simulink model "Final_EWASP_VC"  (R2022a)
settings: Solver=ode1  StartTime=0.0  StopTime=24*3600  FixedStep=10  RelTol=1e-3
values from neighbouring files (symbols this model uses):
  Aux_Threshold = 52    [Setup_Code_EWASP_VC.m]
  buildingAge = 2005    [Setup_Code_EWASP_VC.m]
  ceilingHeight = 2.4    [Setup_Code_EWASP_VC.m]
  conductiveHconnectMatrix = [ ... (first row only)    [Setup_Code_EWASP_VC.m]
  cRoofGreen = 100000    [Setup_Code_EWASP_VC.m]
  Defrost_After_Time = 30    [Setup_Code_EWASP_VC.m]
  DHWDemandProfile = occFreegainHotwaterElecTestPassiveOcc3(:,3)    [Setup_Code_EWASP_VC.m]
  Elec_Max = Elec_Max*(30/24.2)    [Setup_Code_EWASP_VC.m]
  Elec_Mid = Elec_Mid*(30/24.2)    [Setup_Code_EWASP_VC.m]
  Elec_Min = Elec_Min*(30/24.2)    [Setup_Code_EWASP_VC.m]
  ElecDemandProfile = occFreegainHotwaterElecTestPassiveOcc3(:,4)    [Setup_Code_EWASP_VC.m]
  ElecFixed = [Elec_Max(6,2) Elec_Max(6,4) Elec_Max(6,6) Elec_Max(6,7) ... (first row only)    [Setup_Code_EWASP_VC.m]
  floorOrCeilingArea = floorOrCeilingArea*1.15    [Setup_Code_EWASP_VC.m]
  forceCold = 0    [Setup_Code_EWASP_VC.m]
  freegain = occFreegainHotwaterElecTestPassiveOcc3(:,2)-max(occupancy)*25    [Setup_Code_EWASP_VC.m]
  furnitureModelOn = 1    [Setup_Code_EWASP_VC.m]
  Heat_Max = Heat_Max*(30/24.2)    [Setup_Code_EWASP_VC.m]
  Heat_Mid = Heat_Mid*(30/24.2)    [Setup_Code_EWASP_VC.m]
  Heat_Min = Heat_Min*(30/24.2)    [Setup_Code_EWASP_VC.m]
  HeatFixed = [Heat_Max(6,2) Heat_Max(6,4) Heat_Max(6,6) Heat_Max(6,7) ... (first row only)    [Setup_Code_EWASP_VC.m]
  HeatingOnProfile = repmat(HeatingOnProfile,365,1)    [Setup_Code_EWASP_VC.m]
  HEX_ReturnLowerLimit = 52.5    [Setup_Code_EWASP_VC.m]
  HEX_ReturnUpperLimit = 55    [Setup_Code_EWASP_VC.m]
  LeakMultiplier = 1+(2*(rand()-0.5)/10)    [Setup_Code_EWASP_VC.m]
  loopCap = 15    [Setup_Code_EWASP_VC.m]
  maxOcc = max(occupancyProfile)    [Setup_Code_EWASP_VC.m]
  NESW_wallArea = max(NESW_Lengths*ceilingHeight-NESW_Windows,0)    [Setup_Code_EWASP_VC.m]
  NESW_Windows = [ ... (first row only)    [Setup_Code_EWASP_VC.m]
  numRooms = roomCount    [Setup_Code_EWASP_VC.m]
  offsetDays = 0    [Setup_Code_EWASP_VC.m]
  pumpChoice = pumpChoices(MinIndex,1)    [Setup_Code_EWASP_VC.m]
  pumpRamp = 180    [Setup_Code_EWASP_VC.m]
  ReturnLowerLimit = 37.5    [Setup_Code_EWASP_VC.m]
  ReturnUpperLimit = 40    [Setup_Code_EWASP_VC.m]
  RoofIrradiance = Flat_NS_EW_RoofIrradiance(:,1)    [Setup_Code_EWASP_VC.m]
  roofStartTemp = ones(11,1)*20    [Setup_Code_EWASP_VC.m]
  rooftype = 0    [Setup_Code_EWASP_VC.m]
  RoomDataMatrix = [zeros(1,12);ones(1,12)*wallDensity;zeros(1,12);ones(1,12)*wallU;ones(1,12)*windowU;ones(1,12)*floorU;ones(1,12)*ceilingU;zeros(1,12);windowArea, 0;floorOrCeilingArea;zeros(1,12);floorOrCeilingArea*ceilingHeight]    [Setup_Code_EWASP_VC.m]
  roomVol = roomVol*1.15    [Setup_Code_EWASP_VC.m]
  slabStartTemp = (GroundTempTimeSeries(offsetDays*1440+1,1)+thermostatSetting)/2    [Setup_Code_EWASP_VC.m]
  SlackRequest = zeros(1440,1)    [Setup_Code_EWASP_VC.m]
  SolarThermalExists = 0    [Setup_Code_EWASP_VC.m]
  SourceFixed = HeatFixed-ElecFixed    [Setup_Code_EWASP_VC.m]
  StateSeries = StateSeriesGenerator(22,7,1)    [Setup_Code_EWASP_VC.m]
  Tank_Lower_Temp = 49.5    [Setup_Code_EWASP_VC.m]
  Tank_Upper_Temp = 52    [Setup_Code_EWASP_VC.m]
  Tank_Volume_m3 = 0.15    [Setup_Code_EWASP_VC.m]
  TankHeatHour = randi([1 5])-1    [Setup_Code_EWASP_VC.m]
  thermostatSetting = 20.0    (= 20)    [Setup_Code_EWASP_VC.m]
  upDown = [0;0;0;0;1;1;1;1;1;1;1]    [Setup_Code_EWASP_VC.m]
  variableASHP = 1    [Setup_Code_EWASP_VC.m]
  wallStartTempExt = thermostatSetting*(0.266+0.00215*outdoorStartTemp+0.018*wallU+0.00113*outdoorStartTemp*wallU+0.0068*wallU^2)    [Setup_Code_EWASP_VC.m]
undefined symbols (not defined in the file or in its folder): a, ceilingU, condUDMatrix, convUDMatrix, deltaPEXPANDED_E, deltaPEXPANDED_E2, deltaPEXPANDED_N, deltaPEXPANDED_N2, deltaPEXPANDED_S, deltaPEXPANDED_S2, deltaPEXPANDED_W, deltaPEXPANDED_W2, DesiredDHWTemp, DesiredFlowTempVsInOutDeltaTemp, DiffuseHorizontal, DiscIntNeverNeededParam, DNI, dwnAndConcrete, DWORK_A_HX, DWORK_CHK_FLU, DWORK_CP_NODE, DWORK_DH, DWORK_FLUID, DWORK_HCON, DWORK_LOSS, DWORK_MDOTDOWN, DWORK_MDOTIN, DWORK_MDOTUP, DWORK_MIX, DWORK_PRESS, DWORK_QDOTIN, DWORK_RHO_NODE, DWORK_TIN, DWORK_TS_OLD, DWORK_V_NODE, GroundTempTimeSeries, HCM, HCM2, HCM_closed, HCM_closed2, intermediateU, IsTop, massFlowMatrix, neighbourMatrix, numericalRoomUse, RadiatorMatrix, room2roomflowmatrix_E, room2roomflowmatrix_E2, room2roomflowmatrix_N, room2roomflowmatrix_N2, room2roomflowmatrix_S, room2roomflowmatrix_S2, room2roomflowmatrix_W, room2roomflowmatrix_W2, StateAirInEXPANDED_E, StateAirInEXPANDED_E2, StateAirInEXPANDED_N, StateAirInEXPANDED_N2, StateAirInEXPANDED_S, StateAirInEXPANDED_S2 ... (+23)
libraries: simulink x6, dspsigops x4, dspmtrx3 x4, carnot x3, spsEdgeDetectorLib x2, dspstat3 x2, powerlib_meascontrol x1, simulink_extras x1
(part 20 of 27)

== system Final_EWASP_VC/GSHP_Subsystem/Subsystem3/Ground_Source_Heat_Exchanger1/mdot>5 ==
  In1 : Inport
  mdot : Inport  Port=2
  In4 : Inport  Port=3
  Add : Sum
  Fcn2 : Fcn  Expr=u>0
  Fcn3 : Fcn  Expr=u==0
  Product : Product  RndMeth=Zero
  Product1 : Product  RndMeth=Zero
  Out1 : Outport  VectorParamsAs1DForOutWhenUnconnected=off
  wires:
  Fcn3/1 -> Product1/1
  Fcn2/1 -> Product/2
  mdot/1 -> Fcn3/1, Fcn2/1
  In4/1 -> Product1/2
  Add/1 -> Out1/1
  In1/1 -> Product/1
  Product1/1 -> Add/2
  Product/1 -> Add/1

== system Final_EWASP_VC/GSHP_Subsystem/Subsystem3/Ground_Source_Heat_Exchanger1/mdot>6 ==
  In1 : Inport
  mdot : Inport  Port=2
  In4 : Inport  Port=3
  Add : Sum
  Fcn2 : Fcn  Expr=u>0
  Fcn3 : Fcn  Expr=u==0
  Product : Product  RndMeth=Zero
  Product1 : Product  RndMeth=Zero
  Out1 : Outport  VectorParamsAs1DForOutWhenUnconnected=off
  wires:
  Fcn3/1 -> Product1/1
  Fcn2/1 -> Product/2
  mdot/1 -> Fcn3/1, Fcn2/1
  In4/1 -> Product1/2
  Add/1 -> Out1/1
  In1/1 -> Product/1
  Product1/1 -> Add/2
  Product/1 -> Add/1

== system Final_EWASP_VC/GSHP_Subsystem/Subsystem3/Ground_Source_Heat_Exchanger1/mdot>7 ==
  In1 : Inport
  mdot : Inport  Port=2
  In4 : Inport  Port=3
  Add : Sum
  Fcn2 : Fcn  Expr=u>0
  Fcn3 : Fcn  Expr=u==0
  Product : Product  RndMeth=Zero
  Product1 : Product  RndMeth=Zero
  Out1 : Outport  VectorParamsAs1DForOutWhenUnconnected=off
  wires:
  Fcn3/1 -> Product1/1
  Fcn2/1 -> Product/2
  mdot/1 -> Fcn3/1, Fcn2/1
  In4/1 -> Product1/2
  Add/1 -> Out1/1
  In1/1 -> Product/1
  Product1/1 -> Add/2
  Product/1 -> Add/1

== system Final_EWASP_VC/GSHP_Subsystem/Subsystem3/HeatPump_Simplified/HeatPump_basic ==
  Tin_cold : Inport
  Tin_hot : Inport  Port=2
  Tamb : Inport  Port=3
  Ctrl : Inport  Port=4
  mdot_in_cold : Inport  Port=5
  mdot_in_hot : Inport  Port=6
  Ctrl1 : Inport  Port=7
  Bus Creator : BusCreator  Inputs=7
  P_el calculus : Subsystem
  Product : DotProduct  OutDataTypeStr=Inherit: Inherit via internal rule
  Product1 : DotProduct  OutDataTypeStr=Inherit: Inherit via internal rule
  Product3 : DotProduct  OutDataTypeStr=Inherit: Inherit via internal rule
  Sum1 : Sum  Inputs=+-  InputSameDT=on  SaturateOnIntegerOverflow=on  OutDataTypeStr=Inherit: Same as first input
  Sum2 : Sum  Inputs=+-  InputSameDT=on  SaturateOnIntegerOverflow=on  OutDataTypeStr=Inherit: Same as first input
  model cold side : Subsystem
  model hot side : Subsystem
  Tsource : Outport  VectorParamsAs1DForOutWhenUnconnected=off
  THBload : Outport  Port=2  VectorParamsAs1DForOutWhenUnconnected=off
  HPdat : Outport  Port=3  VectorParamsAs1DForOutWhenUnconnected=off
  Real P_Therm : Outport  Port=4  VectorParamsAs1DForOutWhenUnconnected=off
  wires:
  Bus Creator/1 -> HPdat/1
  model hot side/2(Thot_out) -> Bus Creator/5, THBload/1, model cold side/3(Thot), P_el calculus/1(Thot_out), Sum2/1  "Tout_hot"
  Tamb/1 -> model hot side/4(Tamb), model cold side/4(Tamb)
  Tin_hot/1 -> Bus Creator/4, Sum2/2, model hot side/2(Thot)  "THBin_hot"
  mdot_in_hot/1 -> model hot side/3(mdot_hot)
  model hot side/1(mdot*cp) -> Product/1
  Sum2/1 -> Product/2
  Tin_cold/1 -> Bus Creator/1, P_el calculus/2(Tcold_in), model hot side/1(Tcold), Sum1/1, model cold side/1(Tcold)
  model cold side/1(Tcold_out) -> Bus Creator/2, Tsource/1, Sum1/2  "Tcold_out"
  P_el calculus/1(P_el) -> Product1/2
  Product1/1 -> Bus Creator/7  "Pelec"
  Ctrl/1 -> model cold side/5(command), Product1/1, model hot side/5(command)
  mdot_in_cold/1 -> model cold side/2(mdot_cold)
  Sum1/1 -> Product3/1
  model cold side/2(mdot*cp) -> Product3/2
  Product3/1 -> Bus Creator/3  "Qdot_cold"
  Product/1 -> Bus Creator/6  "Qdot_hot"
  model hot side/3(Real P_therm) -> Real P_Therm/1
  Ctrl1/1 -> model hot side/6(Tamb1)

== system Final_EWASP_VC/Subsystem_Room1/Lounge//Dining/Subsystem1/integrate deltat's with initial wall temps as initial condition ==
  In1 : Inport
  In2 : Inport  Port=2
  In3 : Inport  Port=3
  In4 : Inport  Port=4
  Constant : Constant  Value=2
  Constant1 : Constant
  Constant2 : Constant  Value=wallStartTempExt
  Discrete-Time Integrator : DiscreteIntegrator  InitialConditionSource=external  SampleTime=-1  ICPrevOutput=DiscIntNeverNeededParam  ICPrevScaledInput=DiscIntNeverNeededParam
  Discrete-Time Integrator1 : DiscreteIntegrator  InitialConditionSource=external  SampleTime=-1  ICPrevOutput=DiscIntNeverNeededParam  ICPrevScaledInput=DiscIntNeverNeededParam
  Discrete-Time Integrator2 : DiscreteIntegrator  InitialConditionSource=external  SampleTime=-1  ICPrevOutput=DiscIntNeverNeededParam  ICPrevScaledInput=DiscIntNeverNeededParam
  Display : Display
  Divide : Product  Inputs=*/
  Minus1 : Sum
  Minus2 : Sum  Inputs=+-
  Room Initial Temp Table : LookupNDDirect  NumberOfTableDimensions=1  Table=wallStartTempInt'
  Scope{,1..4} (5 alike) : Scope
  Out1 : Outport  VectorParamsAs1DForOutWhenUnconnected=off
  Out2 : Outport  Port=2  VectorParamsAs1DForOutWhenUnconnected=off
  Out3 : Outport  Port=3  VectorParamsAs1DForOutWhenUnconnected=off
  wires:
  Discrete-Time Integrator1/1 -> Scope1/1, Out2/1
  Discrete-Time Integrator2/1 -> Out1/1, Scope/1, Display/1
  Divide/1 -> Discrete-Time Integrator1/2
  In3/1 -> Discrete-Time Integrator/1
  Room Initial Temp Table/1 -> Discrete-Time Integrator2/2, Minus1/1, Scope3/1
  In2/1 -> Discrete-Time Integrator1/1
  Discrete-Time Integrator/1 -> Scope2/1, Out3/1
  Constant2/1 -> Discrete-Time Integrator/2, Minus1/2
  In1/1 -> Discrete-Time Integrator2/1
  In4/1 -> Scope4/1, Minus2/1
  Minus1/1 -> Divide/1
  Constant/1 -> Divide/2
  Constant1/1 -> Minus2/2
  Minus2/1 -> Room Initial Temp Table/1

== system Final_EWASP_VC/Subsystem_Room1/Lounge//Dining/Subsystem2/Irradiance to Solar Gain1 ==
  note: Uses emperical relationship between incidence angle and irradiance through a double glazed window from: ' Simulating Thermochromic and Heat Mirror Glazing Systems in Hot and Cold Climates', G eorgios Kokogiannakis
      |
      | Uses equation for effective diffuse incidence angle from: 'Effective incidence angles of sky-diffuse and ground-reflected irradiance for various incidence angle modifier types', Ehud Strobach. the answer is then multiplied by the diffuse compontent of irradaiance, and also divided by (180-tilt) to account for the fact that only some of the diffuse irradiance is seen by the window (if tilted to 90 o then this is 0.5).
  In1 : Inport
  In2 : Inport  Port=2
  In3 : Inport  Port=3
  In4 : Inport  Port=4
  1-D Lookup Table : Lookup_n-D  NumberOfTableDimensions=1  BreakpointsForDimension1=[0,10,20,30,40,50,60,70,80,90]  Table=[0.53,0.525,0.52,0.51,0.495,0.47,0.415,0.31,0.14,0]  InternalRulePriority=Speed  RndMeth=Simplest
  1-D Lookup Table1 : Lookup_n-D  NumberOfTableDimensions=1  BreakpointsForDimension1=[0,10,20,30,40,50,60,70,80,90]  Table=[0.53,0.525,0.52,0.51,0.495,0.47,0.415,0.31,0.14,0]  InternalRulePriority=Speed  RndMeth=Simplest
  1-D Lookup Table2 : Lookup_n-D  NumberOfTableDimensions=1  BreakpointsForDimension1=[0,10,20,30,40,50,60,70,80,90]  Table=[0.04,0.04,0.04,0.04,0.05,0.05,0.08,0.175,0.38,1]  InternalRulePriority=Speed  RndMeth=Simplest
  1-D Lookup Table3 : Lookup_n-D  NumberOfTableDimensions=1  BreakpointsForDimension1=[0,10,20,30,40,50,60,70,80,90]  Table=[0.04,0.04,0.04,0.04,0.05,0.05,0.08,0.175,0.38,1]  InternalRulePriority=Speed  RndMeth=Simplest
  1-D Lookup Table4 : Lookup_n-D  NumberOfTableDimensions=1  BreakpointsForDimension1=[0,10,20,30,40,50,60,70,80,90]  Table=[0.43,0.435,0.44,0.45,0.455,0.48,0.505,0.515,0.48,0]  InternalRulePriority=Speed  RndMeth=Simplest
  1-D Lookup Table5 : Lookup_n-D  NumberOfTableDimensions=1  BreakpointsForDimension1=[0,10,20,30,40,50,60,70,80,90]  Table=[0.43,0.435,0.44,0.45,0.455,0.48,0.505,0.515,0.48,0]  InternalRulePriority=Speed  RndMeth=Simplest
  Add : Sum
  Add1 : Sum
  Add2 : Sum
  Constant : Constant  Value=180
  Constant1 : Constant  Value=180
  Constant2 : Constant  Value=180
  Fcn1 : Fcn  Expr=59.68-0.1457*u+0.001585*u^2
  Fcn2 : Fcn  Expr=59.68-0.1457*u+0.001585*u^2
  Fcn5 : Fcn  Expr=59.68-0.1457*u+0.001585*u^2
  Product1 : Product  Inputs=*/
  Product2 : Product
  Product3 : Product  Inputs=***
  Product4 : Product
  Product5 : Product  Inputs=*/
  Product6 : Product  Inputs=***
  Product7 : Product
  Product8 : Product  Inputs=***
  Product9 : Product  Inputs=*/
  Reflected portion not currently used : Terminator
  Sum : Sum  Inputs=|+-
  Sum1 : Sum  Inputs=|+-
  Sum2 : Sum  Inputs=|+-
  Out1 : Outport  VectorParamsAs1DForOutWhenUnconnected=off
  Out2 : Outport  Port=2  VectorParamsAs1DForOutWhenUnconnected=off
  wires:
  Product2/1 -> Add/1
  Fcn5/1 -> 1-D Lookup Table1/1
  Product3/1 -> Add/2
  In1/1 -> 1-D Lookup Table4/1, 1-D Lookup Table2/1, 1-D Lookup Table/1
  1-D Lookup Table1/1 -> Product3/1
  1-D Lookup Table/1 -> Product2/1
  Add/1 -> Out1/1
  Constant/1 -> Product1/2, Sum/1
  Sum/1 -> Product1/1
  Product1/1 -> Product3/3
  Product4/1 -> Add1/1
  1-D Lookup Table2/1 -> Product4/1
  In3/1 -> Product7/2, Product4/2, Product2/2
  Product5/1 -> Product6/3
  Constant1/1 -> Product5/2, Sum1/1
  1-D Lookup Table3/1 -> Product6/1
  Sum1/1 -> Product5/1
  Fcn1/1 -> 1-D Lookup Table3/1
  Product6/1 -> Add1/2
  Product7/1 -> Add2/1
  1-D Lookup Table4/1 -> Product7/1
  Product8/1 -> Add2/2
  Sum2/1 -> Product9/1
  Product9/1 -> Product8/3
  Constant2/1 -> Product9/2, Sum2/1
  In4/1 -> Product8/2, Product6/2, Product3/2
  1-D Lookup Table5/1 -> Product8/1
  Fcn2/1 -> 1-D Lookup Table5/1
  In2/1 -> Fcn1/1, Sum1/2, Fcn2/1, Sum2/2, Sum/2, Fcn5/1
  Add1/1 -> Reflected portion not currently used/1
  Add2/1 -> Out2/1

== system Final_EWASP_VC/Subsystem_Room1/Lounge//Dining/Subsystem3/integrate deltat's with initial wall temps as initial condition ==
  In1 : Inport
  In2 : Inport  Port=2
  In3 : Inport  Port=3
  In4 : Inport  Port=4
  Constant : Constant  Value=2
  Constant1 : Constant
  Constant2 : Constant  Value=wallStartTempExt
  Discrete-Time Integrator : DiscreteIntegrator  InitialConditionSource=external  SampleTime=-1  ICPrevOutput=DiscIntNeverNeededParam  ICPrevScaledInput=DiscIntNeverNeededParam
  Discrete-Time Integrator1 : DiscreteIntegrator  InitialConditionSource=external  SampleTime=-1  ICPrevOutput=DiscIntNeverNeededParam  ICPrevScaledInput=DiscIntNeverNeededParam
  Discrete-Time Integrator2 : DiscreteIntegrator  InitialConditionSource=external  SampleTime=-1  ICPrevOutput=DiscIntNeverNeededParam  ICPrevScaledInput=DiscIntNeverNeededParam
  Display : Display
  Divide : Product  Inputs=*/
  Minus1 : Sum
  Minus2 : Sum  Inputs=+-
  Room Initial Temp Table : LookupNDDirect  NumberOfTableDimensions=1  Table=roofStartTemp
  Scope{,1..2,4} (4 alike) : Scope
  Out1 : Outport  VectorParamsAs1DForOutWhenUnconnected=off
  Out2 : Outport  Port=2  VectorParamsAs1DForOutWhenUnconnected=off
  Out3 : Outport  Port=3  VectorParamsAs1DForOutWhenUnconnected=off
  wires:
  Discrete-Time Integrator1/1 -> Scope1/1, Out2/1
  Discrete-Time Integrator2/1 -> Out1/1, Scope/1, Display/1
  Divide/1 -> Discrete-Time Integrator1/2
  In3/1 -> Discrete-Time Integrator/1
  Room Initial Temp Table/1 -> Discrete-Time Integrator2/2, Minus1/1
  In2/1 -> Discrete-Time Integrator1/1
  Discrete-Time Integrator/1 -> Scope2/1, Out3/1
  Constant2/1 -> Discrete-Time Integrator/2, Minus1/2
  In1/1 -> Discrete-Time Integrator2/1
  In4/1 -> Scope4/1, Minus2/1
  Minus1/1 -> Divide/1
  Constant/1 -> Divide/2
  Constant1/1 -> Minus2/2
  Minus2/1 -> Room Initial Temp Table/1

== system Final_EWASP_VC/Subsystem_Room1/Lounge//Dining/Subsystem6/integrate deltat's with initial wall temps as initial condition ==
  In1 : Inport
  In2 : Inport  Port=2
  In3 : Inport  Port=3
  In5 : Inport  Port=4
  In6 : Inport  Port=5
  In7 : Inport  Port=6
  In8 : Inport  Port=7
  In9 : Inport  Port=8
  In4 : Inport  Port=9
  In11 : Inport  Port=10
  Constant{,3..4,7,10..11,14..15,18..19,22..23,26..27} (14 alike) : Constant  Value=8
  Constant1 : Constant
  Constant12 : Constant  Value=5
  Constant13 : Constant  Value=3
  Constant16 : Constant  Value=4
  Constant17 : Constant  Value=4
  Constant2 : Constant  Value=wallStartTempExt
  Constant20 : Constant  Value=3
  Constant21 : Constant  Value=5
  Constant24 : Constant  Value=2
  Constant25 : Constant  Value=6
  Constant28 : Constant
  Constant29 : Constant  Value=7
  Constant5 : Constant  Value=7
  Constant6 : Constant
  Constant8 : Constant  Value=6
  Constant9 : Constant  Value=2
  Discrete-Time Integrator{,1..8} (9 alike) : DiscreteIntegrator  InitialConditionSource=external  SampleTime=-1  ICPrevOutput=DiscIntNeverNeededParam  ICPrevScaledInput=DiscIntNeverNeededParam
  Display : Display
  Divide{,1..13} (14 alike) : Product  Inputs=*/*
  Minus{1,3..8} (7 alike) : Sum
  Minus2 : Sum  Inputs=+-
  Room Initial Temp Table : LookupNDDirect  NumberOfTableDimensions=1  Table=wallStartTempInt'
  Scope{,1,3..4} (4 alike) : Scope
  Out1 : Outport  VectorParamsAs1DForOutWhenUnconnected=off
  Out2 : Outport  Port=2  VectorParamsAs1DForOutWhenUnconnected=off
  Out3 : Outport  Port=3  VectorParamsAs1DForOutWhenUnconnected=off
  Out4 : Outport  Port=4  VectorParamsAs1DForOutWhenUnconnected=off
  Out5 : Outport  Port=5  VectorParamsAs1DForOutWhenUnconnected=off
  Out6 : Outport  Port=6  VectorParamsAs1DForOutWhenUnconnected=off
  Out7 : Outport  Port=7  VectorParamsAs1DForOutWhenUnconnected=off
  Out8 : Outport  Port=8  VectorParamsAs1DForOutWhenUnconnected=off
  Out10 : Outport  Port=9  VectorParamsAs1DForOutWhenUnconnected=off
  wires:
  Discrete-Time Integrator1/1 -> Scope1/1, Out2/1
  Discrete-Time Integrator2/1 -> Out1/1, Scope/1, Display/1
  Room Initial Temp Table/1 -> [int], Scope3/1
  In2/1 -> Discrete-Time Integrator1/1
  Constant2/1 -> [ext]
  In1/1 -> Discrete-Time Integrator2/1
  In11/1 -> Scope4/1, Minus2/1
  Constant1/1 -> Minus2/2
  Minus2/1 -> Room Initial Temp Table/1
  [int] -> Discrete-Time Integrator2/2
  [ext] -> Discrete-Time Integrator/2
  Divide/1 -> Minus1/1
  Divide1/1 -> Minus1/2
  Constant/1 -> Divide/2
  Constant4/1 -> Divide1/2
  [int] -> Divide/1
  [ext] -> Divide1/1
  Constant5/1 -> Divide/3
  Constant6/1 -> Divide1/3
  Minus1/1 -> Discrete-Time Integrator1/2
  Minus3/1 -> Discrete-Time Integrator3/2
  Constant9/1 -> Divide3/3
  [ext] -> Divide3/1
  Constant8/1 -> Divide2/3
  [int] -> Divide2/1
  Constant7/1 -> Divide3/2
  Constant3/1 -> Divide2/2
  Divide3/1 -> Minus3/2
  Divide2/1 -> Minus3/1
  Minus4/1 -> Discrete-Time Integrator4/2
  Constant13/1 -> Divide5/3
  [ext] -> Divide5/1
  Constant12/1 -> Divide4/3
  [int] -> Divide4/1
  Constant11/1 -> Divide5/2
  Constant10/1 -> Divide4/2
  Divide5/1 -> Minus4/2
  Divide4/1 -> Minus4/1
  Minus5/1 -> Discrete-Time Integrator5/2
  Constant17/1 -> Divide7/3
  [ext] -> Divide7/1
  Constant16/1 -> Divide6/3
  [int] -> Divide6/1
  Constant15/1 -> Divide7/2
  Constant14/1 -> Divide6/2
  Divide7/1 -> Minus5/2
  Divide6/1 -> Minus5/1
  In3/1 -> Discrete-Time Integrator3/1
  In5/1 -> Discrete-Time Integrator4/1
  In6/1 -> Discrete-Time Integrator5/1
  Divide8/1 -> Minus6/1
  Constant19/1 -> Divide9/2
  Constant18/1 -> Divide8/2
  Divide9/1 -> Minus6/2
  [ext] -> Divide9/1
  Constant21/1 -> Divide9/3
  Minus6/1 -> Discrete-Time Integrator6/2
  Constant20/1 -> Divide8/3
  [int] -> Divide8/1
  Divide10/1 -> Minus7/1
  Constant23/1 -> Divide11/2
  Constant22/1 -> Divide10/2
  Divide11/1 -> Minus7/2
  [ext] -> Divide11/1
  Constant25/1 -> Divide11/3
  Minus7/1 -> Discrete-Time Integrator7/2
  Constant24/1 -> Divide10/3
  [int] -> Divide10/1
  Divide12/1 -> Minus8/1
  Constant27/1 -> Divide13/2
  Constant26/1 -> Divide12/2
  Divide13/1 -> Minus8/2
  [ext] -> Divide13/1
  Constant29/1 -> Divide13/3
  Minus8/1 -> Discrete-Time Integrator8/2
  Constant28/1 -> Divide12/3
  [int] -> Divide12/1
  In7/1 -> Discrete-Time Integrator6/1
  In8/1 -> Discrete-Time Integrator7/1
  In9/1 -> Discrete-Time Integrator8/1
  Discrete-Time Integrator3/1 -> Out3/1
  Discrete-Time Integrator4/1 -> Out4/1
  Discrete-Time Integrator5/1 -> Out5/1
  Discrete-Time Integrator6/1 -> Out6/1
  Discrete-Time Integrator7/1 -> Out7/1
  Discrete-Time Integrator8/1 -> Out8/1
  Discrete-Time Integrator/1 -> Out10/1
  In4/1 -> Discrete-Time Integrator/1

== system Final_EWASP_VC/Subsystem_Room10/En suite/Subsystem1/integrate deltat's with initial wall temps as initial condition ==
  In1 : Inport
  In2 : Inport  Port=2
  In3 : Inport  Port=3
  In4 : Inport  Port=4
  Constant : Constant  Value=2
  Constant1 : Constant
  Constant2 : Constant  Value=wallStartTempExt
  Discrete-Time Integrator : DiscreteIntegrator  InitialConditionSource=external  SampleTime=-1  ICPrevOutput=DiscIntNeverNeededParam  ICPrevScaledInput=DiscIntNeverNeededParam
  Discrete-Time Integrator1 : DiscreteIntegrator  InitialConditionSource=external  SampleTime=-1  ICPrevOutput=DiscIntNeverNeededParam  ICPrevScaledInput=DiscIntNeverNeededParam
  Discrete-Time Integrator2 : DiscreteIntegrator  InitialConditionSource=external  SampleTime=-1  ICPrevOutput=DiscIntNeverNeededParam  ICPrevScaledInput=DiscIntNeverNeededParam
  Display : Display
  Divide : Product  Inputs=*/
  Minus1 : Sum
  Minus2 : Sum  Inputs=+-
  Room Initial Temp Table : LookupNDDirect  NumberOfTableDimensions=1  Table=wallStartTempInt'
  Scope{,1..4} (5 alike) : Scope
  Out1 : Outport  VectorParamsAs1DForOutWhenUnconnected=off
  Out2 : Outport  Port=2  VectorParamsAs1DForOutWhenUnconnected=off
  Out3 : Outport  Port=3  VectorParamsAs1DForOutWhenUnconnected=off
  wires:
  Discrete-Time Integrator1/1 -> Scope1/1, Out2/1
  Discrete-Time Integrator2/1 -> Out1/1, Scope/1, Display/1
  Divide/1 -> Discrete-Time Integrator1/2
  In3/1 -> Discrete-Time Integrator/1
  Room Initial Temp Table/1 -> Discrete-Time Integrator2/2, Minus1/1, Scope3/1
  In2/1 -> Discrete-Time Integrator1/1
  Discrete-Time Integrator/1 -> Scope2/1, Out3/1
  Constant2/1 -> Discrete-Time Integrator/2, Minus1/2
  In1/1 -> Discrete-Time Integrator2/1
  In4/1 -> Scope4/1, Minus2/1
  Minus1/1 -> Divide/1
  Constant/1 -> Divide/2
  Constant1/1 -> Minus2/2
  Minus2/1 -> Room Initial Temp Table/1

== system Final_EWASP_VC/Subsystem_Room10/En suite/Subsystem3/integrate deltat's with initial wall temps as initial condition ==
  In1 : Inport
  In2 : Inport  Port=2
  In3 : Inport  Port=3
  In4 : Inport  Port=4
  Constant : Constant  Value=2
  Constant1 : Constant
  Constant2 : Constant  Value=wallStartTempExt
  Discrete-Time Integrator : DiscreteIntegrator  InitialConditionSource=external  SampleTime=-1  ICPrevOutput=DiscIntNeverNeededParam  ICPrevScaledInput=DiscIntNeverNeededParam
  Discrete-Time Integrator1 : DiscreteIntegrator  InitialConditionSource=external  SampleTime=-1  ICPrevOutput=DiscIntNeverNeededParam  ICPrevScaledInput=DiscIntNeverNeededParam
  Discrete-Time Integrator2 : DiscreteIntegrator  InitialConditionSource=external  SampleTime=-1  ICPrevOutput=DiscIntNeverNeededParam  ICPrevScaledInput=DiscIntNeverNeededParam
  Display : Display
  Divide : Product  Inputs=*/
  Minus1 : Sum
  Minus2 : Sum  Inputs=+-
  Room Initial Temp Table : LookupNDDirect  NumberOfTableDimensions=1  Table=roofStartTemp
  Scope{,1..2,4} (4 alike) : Scope
  Out1 : Outport  VectorParamsAs1DForOutWhenUnconnected=off
  Out2 : Outport  Port=2  VectorParamsAs1DForOutWhenUnconnected=off
  Out3 : Outport  Port=3  VectorParamsAs1DForOutWhenUnconnected=off
  wires:
  Discrete-Time Integrator1/1 -> Scope1/1, Out2/1
  Discrete-Time Integrator2/1 -> Out1/1, Scope/1, Display/1
  Divide/1 -> Discrete-Time Integrator1/2
  In3/1 -> Discrete-Time Integrator/1
  Room Initial Temp Table/1 -> Discrete-Time Integrator2/2, Minus1/1
  In2/1 -> Discrete-Time Integrator1/1
  Discrete-Time Integrator/1 -> Scope2/1, Out3/1
  Constant2/1 -> Discrete-Time Integrator/2, Minus1/2
  In1/1 -> Discrete-Time Integrator2/1
  In4/1 -> Scope4/1, Minus2/1
  Minus1/1 -> Divide/1
  Constant/1 -> Divide/2
  Constant1/1 -> Minus2/2
  Minus2/1 -> Room Initial Temp Table/1

== system Final_EWASP_VC/Subsystem_Room10/En suite/Subsystem4/Irradiance to Solar Gain1 ==
  note: Uses emperical relationship between incidence angle and irradiance through a double glazed window from: ' Simulating Thermochromic and Heat Mirror Glazing Systems in Hot and Cold Climates', G eorgios Kokogiannakis
      |
      | Uses equation for effective diffuse incidence angle from: 'Effective incidence angles of sky-diffuse and ground-reflected irradiance for various incidence angle modifier types', Ehud Strobach. the answer is then multiplied by the diffuse compontent of irradaiance, and also divided by (180-tilt) to account for the fact that only some of the diffuse irradiance is seen by the window (if tilted to 90 o then this is 0.5).
  In1 : Inport
  In2 : Inport  Port=2
  In3 : Inport  Port=3
  In4 : Inport  Port=4
  1-D Lookup Table : Lookup_n-D  NumberOfTableDimensions=1  BreakpointsForDimension1=[0,10,20,30,40,50,60,70,80,90]  Table=[0.53,0.525,0.52,0.51,0.495,0.47,0.415,0.31,0.14,0]  InternalRulePriority=Speed  RndMeth=Simplest
  1-D Lookup Table1 : Lookup_n-D  NumberOfTableDimensions=1  BreakpointsForDimension1=[0,10,20,30,40,50,60,70,80,90]  Table=[0.53,0.525,0.52,0.51,0.495,0.47,0.415,0.31,0.14,0]  InternalRulePriority=Speed  RndMeth=Simplest
  1-D Lookup Table2 : Lookup_n-D  NumberOfTableDimensions=1  BreakpointsForDimension1=[0,10,20,30,40,50,60,70,80,90]  Table=[0.04,0.04,0.04,0.04,0.05,0.05,0.08,0.175,0.38,1]  InternalRulePriority=Speed  RndMeth=Simplest
  1-D Lookup Table3 : Lookup_n-D  NumberOfTableDimensions=1  BreakpointsForDimension1=[0,10,20,30,40,50,60,70,80,90]  Table=[0.04,0.04,0.04,0.04,0.05,0.05,0.08,0.175,0.38,1]  InternalRulePriority=Speed  RndMeth=Simplest
  1-D Lookup Table4 : Lookup_n-D  NumberOfTableDimensions=1  BreakpointsForDimension1=[0,10,20,30,40,50,60,70,80,90]  Table=[0.43,0.435,0.44,0.45,0.455,0.48,0.505,0.515,0.48,0]  InternalRulePriority=Speed  RndMeth=Simplest
  1-D Lookup Table5 : Lookup_n-D  NumberOfTableDimensions=1  BreakpointsForDimension1=[0,10,20,30,40,50,60,70,80,90]  Table=[0.43,0.435,0.44,0.45,0.455,0.48,0.505,0.515,0.48,0]  InternalRulePriority=Speed  RndMeth=Simplest
  Add : Sum
  Add1 : Sum
  Add2 : Sum
  Constant : Constant  Value=180
  Constant1 : Constant  Value=180
  Constant2 : Constant  Value=180
  Fcn1 : Fcn  Expr=59.68-0.1457*u+0.001585*u^2
  Fcn2 : Fcn  Expr=59.68-0.1457*u+0.001585*u^2
  Fcn5 : Fcn  Expr=59.68-0.1457*u+0.001585*u^2
  Product1 : Product  Inputs=*/
  Product2 : Product
  Product3 : Product  Inputs=***
  Product4 : Product
  Product5 : Product  Inputs=*/
  Product6 : Product  Inputs=***
  Product7 : Product
  Product8 : Product  Inputs=***
  Product9 : Product  Inputs=*/
  Reflected portion not currently used : Terminator
  Sum : Sum  Inputs=|+-
  Sum1 : Sum  Inputs=|+-
  Sum2 : Sum  Inputs=|+-
  Out1 : Outport  VectorParamsAs1DForOutWhenUnconnected=off
  Out2 : Outport  Port=2  VectorParamsAs1DForOutWhenUnconnected=off
  wires:
  Product2/1 -> Add/1
  Fcn5/1 -> 1-D Lookup Table1/1
  Product3/1 -> Add/2
  In1/1 -> 1-D Lookup Table4/1, 1-D Lookup Table2/1, 1-D Lookup Table/1
  1-D Lookup Table1/1 -> Product3/1
  1-D Lookup Table/1 -> Product2/1
  Add/1 -> Out1/1
  Constant/1 -> Product1/2, Sum/1
  Sum/1 -> Product1/1
  Product1/1 -> Product3/3
  Product4/1 -> Add1/1
  1-D Lookup Table2/1 -> Product4/1
  In3/1 -> Product7/2, Product4/2, Product2/2
  Product5/1 -> Product6/3
  Constant1/1 -> Product5/2, Sum1/1
  1-D Lookup Table3/1 -> Product6/1
  Sum1/1 -> Product5/1
  Fcn1/1 -> 1-D Lookup Table3/1
  Product6/1 -> Add1/2
  Product7/1 -> Add2/1
  1-D Lookup Table4/1 -> Product7/1
  Product8/1 -> Add2/2
  Sum2/1 -> Product9/1
  Product9/1 -> Product8/3
  Constant2/1 -> Product9/2, Sum2/1
  In4/1 -> Product8/2, Product6/2, Product3/2
  1-D Lookup Table5/1 -> Product8/1
  Fcn2/1 -> 1-D Lookup Table5/1
  In2/1 -> Fcn1/1, Sum1/2, Fcn2/1, Sum2/2, Sum/2, Fcn5/1
  Add1/1 -> Reflected portion not currently used/1
  Add2/1 -> Out2/1

== system Final_EWASP_VC/Subsystem_Room11/Bathroom/Subsystem1/integrate deltat's with initial wall temps as initial condition ==
  In1 : Inport
  In2 : Inport  Port=2
  In3 : Inport  Port=3
  In4 : Inport  Port=4
  Constant : Constant  Value=2
  Constant1 : Constant
  Constant2 : Constant  Value=wallStartTempExt
  Discrete-Time Integrator : DiscreteIntegrator  InitialConditionSource=external  SampleTime=-1  ICPrevOutput=DiscIntNeverNeededParam  ICPrevScaledInput=DiscIntNeverNeededParam
  Discrete-Time Integrator1 : DiscreteIntegrator  InitialConditionSource=external  SampleTime=-1  ICPrevOutput=DiscIntNeverNeededParam  ICPrevScaledInput=DiscIntNeverNeededParam
  Discrete-Time Integrator2 : DiscreteIntegrator  InitialConditionSource=external  SampleTime=-1  ICPrevOutput=DiscIntNeverNeededParam  ICPrevScaledInput=DiscIntNeverNeededParam
  Display : Display
  Divide : Product  Inputs=*/
  Minus1 : Sum
  Minus2 : Sum  Inputs=+-
  Room Initial Temp Table : LookupNDDirect  NumberOfTableDimensions=1  Table=wallStartTempInt'
  Scope{,1..4} (5 alike) : Scope
  Out1 : Outport  VectorParamsAs1DForOutWhenUnconnected=off
  Out2 : Outport  Port=2  VectorParamsAs1DForOutWhenUnconnected=off
  Out3 : Outport  Port=3  VectorParamsAs1DForOutWhenUnconnected=off
  wires:
  Discrete-Time Integrator1/1 -> Scope1/1, Out2/1
  Discrete-Time Integrator2/1 -> Out1/1, Scope/1, Display/1
  Divide/1 -> Discrete-Time Integrator1/2
  In3/1 -> Discrete-Time Integrator/1
  Room Initial Temp Table/1 -> Discrete-Time Integrator2/2, Minus1/1, Scope3/1
  In2/1 -> Discrete-Time Integrator1/1
  Discrete-Time Integrator/1 -> Scope2/1, Out3/1
  Constant2/1 -> Discrete-Time Integrator/2, Minus1/2
  In1/1 -> Discrete-Time Integrator2/1
  In4/1 -> Scope4/1, Minus2/1
  Minus1/1 -> Divide/1
  Constant/1 -> Divide/2
  Constant1/1 -> Minus2/2
  Minus2/1 -> Room Initial Temp Table/1

== system Final_EWASP_VC/Subsystem_Room11/Bathroom/Subsystem2/Irradiance to Solar Gain1 ==
  note: Uses emperical relationship between incidence angle and irradiance through a double glazed window from: ' Simulating Thermochromic and Heat Mirror Glazing Systems in Hot and Cold Climates', G eorgios Kokogiannakis
      |
      | Uses equation for effective diffuse incidence angle from: 'Effective incidence angles of sky-diffuse and ground-reflected irradiance for various incidence angle modifier types', Ehud Strobach. the answer is then multiplied by the diffuse compontent of irradaiance, and also divided by (180-tilt) to account for the fact that only some of the diffuse irradiance is seen by the window (if tilted to 90 o then this is 0.5).
  In1 : Inport
  In2 : Inport  Port=2
  In3 : Inport  Port=3
  In4 : Inport  Port=4
  1-D Lookup Table : Lookup_n-D  NumberOfTableDimensions=1  BreakpointsForDimension1=[0,10,20,30,40,50,60,70,80,90]  Table=[0.53,0.525,0.52,0.51,0.495,0.47,0.415,0.31,0.14,0]  InternalRulePriority=Speed  RndMeth=Simplest
  1-D Lookup Table1 : Lookup_n-D  NumberOfTableDimensions=1  BreakpointsForDimension1=[0,10,20,30,40,50,60,70,80,90]  Table=[0.53,0.525,0.52,0.51,0.495,0.47,0.415,0.31,0.14,0]  InternalRulePriority=Speed  RndMeth=Simplest
  1-D Lookup Table2 : Lookup_n-D  NumberOfTableDimensions=1  BreakpointsForDimension1=[0,10,20,30,40,50,60,70,80,90]  Table=[0.04,0.04,0.04,0.04,0.05,0.05,0.08,0.175,0.38,1]  InternalRulePriority=Speed  RndMeth=Simplest
  1-D Lookup Table3 : Lookup_n-D  NumberOfTableDimensions=1  BreakpointsForDimension1=[0,10,20,30,40,50,60,70,80,90]  Table=[0.04,0.04,0.04,0.04,0.05,0.05,0.08,0.175,0.38,1]  InternalRulePriority=Speed  RndMeth=Simplest
  1-D Lookup Table4 : Lookup_n-D  NumberOfTableDimensions=1  BreakpointsForDimension1=[0,10,20,30,40,50,60,70,80,90]  Table=[0.43,0.435,0.44,0.45,0.455,0.48,0.505,0.515,0.48,0]  InternalRulePriority=Speed  RndMeth=Simplest
  1-D Lookup Table5 : Lookup_n-D  NumberOfTableDimensions=1  BreakpointsForDimension1=[0,10,20,30,40,50,60,70,80,90]  Table=[0.43,0.435,0.44,0.45,0.455,0.48,0.505,0.515,0.48,0]  InternalRulePriority=Speed  RndMeth=Simplest
  Add : Sum
  Add1 : Sum
  Add2 : Sum
  Constant : Constant  Value=180
  Constant1 : Constant  Value=180
  Constant2 : Constant  Value=180
  Fcn1 : Fcn  Expr=59.68-0.1457*u+0.001585*u^2
  Fcn2 : Fcn  Expr=59.68-0.1457*u+0.001585*u^2
  Fcn5 : Fcn  Expr=59.68-0.1457*u+0.001585*u^2
  Product1 : Product  Inputs=*/
  Product2 : Product
  Product3 : Product  Inputs=***
  Product4 : Product
  Product5 : Product  Inputs=*/
  Product6 : Product  Inputs=***
  Product7 : Product
  Product8 : Product  Inputs=***
  Product9 : Product  Inputs=*/
  Reflected portion not currently used : Terminator
  Sum : Sum  Inputs=|+-
  Sum1 : Sum  Inputs=|+-
  Sum2 : Sum  Inputs=|+-
  Out1 : Outport  VectorParamsAs1DForOutWhenUnconnected=off
  Out2 : Outport  Port=2  VectorParamsAs1DForOutWhenUnconnected=off
  wires:
  Product2/1 -> Add/1
  Fcn5/1 -> 1-D Lookup Table1/1
  Product3/1 -> Add/2
  In1/1 -> 1-D Lookup Table4/1, 1-D Lookup Table2/1, 1-D Lookup Table/1
  1-D Lookup Table1/1 -> Product3/1
  1-D Lookup Table/1 -> Product2/1
  Add/1 -> Out1/1
  Constant/1 -> Product1/2, Sum/1
  Sum/1 -> Product1/1
  Product1/1 -> Product3/3
  Product4/1 -> Add1/1
  1-D Lookup Table2/1 -> Product4/1
  In3/1 -> Product7/2, Product4/2, Product2/2
  Product5/1 -> Product6/3
  Constant1/1 -> Product5/2, Sum1/1
  1-D Lookup Table3/1 -> Product6/1
  Sum1/1 -> Product5/1
  Fcn1/1 -> 1-D Lookup Table3/1
  Product6/1 -> Add1/2
  Product7/1 -> Add2/1
  1-D Lookup Table4/1 -> Product7/1
  Product8/1 -> Add2/2
  Sum2/1 -> Product9/1
  Product9/1 -> Product8/3
  Constant2/1 -> Product9/2, Sum2/1
  In4/1 -> Product8/2, Product6/2, Product3/2
  1-D Lookup Table5/1 -> Product8/1
  Fcn2/1 -> 1-D Lookup Table5/1
  In2/1 -> Fcn1/1, Sum1/2, Fcn2/1, Sum2/2, Sum/2, Fcn5/1
  Add1/1 -> Reflected portion not currently used/1
  Add2/1 -> Out2/1

== system Final_EWASP_VC/Subsystem_Room11/Bathroom/Subsystem3/integrate deltat's with initial wall temps as initial condition ==
  In1 : Inport
  In2 : Inport  Port=2
  In3 : Inport  Port=3
  In4 : Inport  Port=4
  Constant : Constant  Value=2
  Constant1 : Constant
  Constant2 : Constant  Value=wallStartTempExt
  Discrete-Time Integrator : DiscreteIntegrator  InitialConditionSource=external  SampleTime=-1  ICPrevOutput=DiscIntNeverNeededParam  ICPrevScaledInput=DiscIntNeverNeededParam
  Discrete-Time Integrator1 : DiscreteIntegrator  InitialConditionSource=external  SampleTime=-1  ICPrevOutput=DiscIntNeverNeededParam  ICPrevScaledInput=DiscIntNeverNeededParam
  Discrete-Time Integrator2 : DiscreteIntegrator  InitialConditionSource=external  SampleTime=-1  ICPrevOutput=DiscIntNeverNeededParam  ICPrevScaledInput=DiscIntNeverNeededParam
  Display : Display
  Divide : Product  Inputs=*/
  Minus1 : Sum
  Minus2 : Sum  Inputs=+-
  Room Initial Temp Table : LookupNDDirect  NumberOfTableDimensions=1  Table=roofStartTemp
  Scope{,1..2,4} (4 alike) : Scope
  Out1 : Outport  VectorParamsAs1DForOutWhenUnconnected=off
  Out2 : Outport  Port=2  VectorParamsAs1DForOutWhenUnconnected=off
  Out3 : Outport  Port=3  VectorParamsAs1DForOutWhenUnconnected=off
  wires:
  Discrete-Time Integrator1/1 -> Scope1/1, Out2/1
  Discrete-Time Integrator2/1 -> Out1/1, Scope/1, Display/1
  Divide/1 -> Discrete-Time Integrator1/2
  In3/1 -> Discrete-Time Integrator/1
  Room Initial Temp Table/1 -> Discrete-Time Integrator2/2, Minus1/1
  In2/1 -> Discrete-Time Integrator1/1
  Discrete-Time Integrator/1 -> Scope2/1, Out3/1
  Constant2/1 -> Discrete-Time Integrator/2, Minus1/2
  In1/1 -> Discrete-Time Integrator2/1
  In4/1 -> Scope4/1, Minus2/1
  Minus1/1 -> Divide/1
  Constant/1 -> Divide/2
  Constant1/1 -> Minus2/2
  Minus2/1 -> Room Initial Temp Table/1

== system Final_EWASP_VC/Subsystem_Room2/Kitchen/Subsystem1/integrate deltat's with initial wall temps as initial condition ==
  In1 : Inport
  In2 : Inport  Port=2
  In3 : Inport  Port=3
  In4 : Inport  Port=4
  Constant : Constant  Value=2
  Constant1 : Constant
  Constant2 : Constant  Value=wallStartTempExt
  Discrete-Time Integrator : DiscreteIntegrator  InitialConditionSource=external  SampleTime=-1  ICPrevOutput=DiscIntNeverNeededParam  ICPrevScaledInput=DiscIntNeverNeededParam
  Discrete-Time Integrator1 : DiscreteIntegrator  InitialConditionSource=external  SampleTime=-1  ICPrevOutput=DiscIntNeverNeededParam  ICPrevScaledInput=DiscIntNeverNeededParam
  Discrete-Time Integrator2 : DiscreteIntegrator  InitialConditionSource=external  SampleTime=-1  ICPrevOutput=DiscIntNeverNeededParam  ICPrevScaledInput=DiscIntNeverNeededParam
  Display : Display
  Divide : Product  Inputs=*/
  Minus1 : Sum
  Minus2 : Sum  Inputs=+-
  Room Initial Temp Table : LookupNDDirect  NumberOfTableDimensions=1  Table=wallStartTempInt'
  Scope{,1..4} (5 alike) : Scope
  Out1 : Outport  VectorParamsAs1DForOutWhenUnconnected=off
  Out2 : Outport  Port=2  VectorParamsAs1DForOutWhenUnconnected=off
  Out3 : Outport  Port=3  VectorParamsAs1DForOutWhenUnconnected=off
  wires:
  Discrete-Time Integrator1/1 -> Scope1/1, Out2/1
  Discrete-Time Integrator2/1 -> Out1/1, Scope/1, Display/1
  Divide/1 -> Discrete-Time Integrator1/2
  In3/1 -> Discrete-Time Integrator/1
  Room Initial Temp Table/1 -> Discrete-Time Integrator2/2, Minus1/1, Scope3/1
  In2/1 -> Discrete-Time Integrator1/1
  Discrete-Time Integrator/1 -> Scope2/1, Out3/1
  Constant2/1 -> Discrete-Time Integrator/2, Minus1/2
  In1/1 -> Discrete-Time Integrator2/1
  In4/1 -> Scope4/1, Minus2/1
  Minus1/1 -> Divide/1
  Constant/1 -> Divide/2
  Constant1/1 -> Minus2/2
  Minus2/1 -> Room Initial Temp Table/1

== system Final_EWASP_VC/Subsystem_Room2/Kitchen/Subsystem3/integrate deltat's with initial wall temps as initial condition ==
  In1 : Inport
  In2 : Inport  Port=2
  In3 : Inport  Port=3
  In4 : Inport  Port=4
  Constant : Constant  Value=2
  Constant1 : Constant
  Constant2 : Constant  Value=wallStartTempExt
  Discrete-Time Integrator : DiscreteIntegrator  InitialConditionSource=external  SampleTime=-1  ICPrevOutput=DiscIntNeverNeededParam  ICPrevScaledInput=DiscIntNeverNeededParam
  Discrete-Time Integrator1 : DiscreteIntegrator  InitialConditionSource=external  SampleTime=-1  ICPrevOutput=DiscIntNeverNeededParam  ICPrevScaledInput=DiscIntNeverNeededParam
  Discrete-Time Integrator2 : DiscreteIntegrator  InitialConditionSource=external  SampleTime=-1  ICPrevOutput=DiscIntNeverNeededParam  ICPrevScaledInput=DiscIntNeverNeededParam
  Display : Display
  Divide : Product  Inputs=*/
  Minus1 : Sum
  Minus2 : Sum  Inputs=+-
  Room Initial Temp Table : LookupNDDirect  NumberOfTableDimensions=1  Table=roofStartTemp
  Scope{,1..2,4} (4 alike) : Scope
  Out1 : Outport  VectorParamsAs1DForOutWhenUnconnected=off
  Out2 : Outport  Port=2  VectorParamsAs1DForOutWhenUnconnected=off
  Out3 : Outport  Port=3  VectorParamsAs1DForOutWhenUnconnected=off
  wires:
  Discrete-Time Integrator1/1 -> Scope1/1, Out2/1
  Discrete-Time Integrator2/1 -> Out1/1, Scope/1, Display/1
  Divide/1 -> Discrete-Time Integrator1/2
  In3/1 -> Discrete-Time Integrator/1
  Room Initial Temp Table/1 -> Discrete-Time Integrator2/2, Minus1/1
  In2/1 -> Discrete-Time Integrator1/1
  Discrete-Time Integrator/1 -> Scope2/1, Out3/1
  Constant2/1 -> Discrete-Time Integrator/2, Minus1/2
  In1/1 -> Discrete-Time Integrator2/1
  In4/1 -> Scope4/1, Minus2/1
  Minus1/1 -> Divide/1
  Constant/1 -> Divide/2
  Constant1/1 -> Minus2/2
  Minus2/1 -> Room Initial Temp Table/1

== system Final_EWASP_VC/Subsystem_Room2/Kitchen/Subsystem4/Irradiance to Solar Gain1 ==
  note: Uses emperical relationship between incidence angle and irradiance through a double glazed window from: ' Simulating Thermochromic and Heat Mirror Glazing Systems in Hot and Cold Climates', G eorgios Kokogiannakis
      |
      | Uses equation for effective diffuse incidence angle from: 'Effective incidence angles of sky-diffuse and ground-reflected irradiance for various incidence angle modifier types', Ehud Strobach. the answer is then multiplied by the diffuse compontent of irradaiance, and also divided by (180-tilt) to account for the fact that only some of the diffuse irradiance is seen by the window (if tilted to 90 o then this is 0.5).
  In1 : Inport
  In2 : Inport  Port=2
  In3 : Inport  Port=3
  In4 : Inport  Port=4
  1-D Lookup Table : Lookup_n-D  NumberOfTableDimensions=1  BreakpointsForDimension1=[0,10,20,30,40,50,60,70,80,90]  Table=[0.53,0.525,0.52,0.51,0.495,0.47,0.415,0.31,0.14,0]  InternalRulePriority=Speed  RndMeth=Simplest
  1-D Lookup Table1 : Lookup_n-D  NumberOfTableDimensions=1  BreakpointsForDimension1=[0,10,20,30,40,50,60,70,80,90]  Table=[0.53,0.525,0.52,0.51,0.495,0.47,0.415,0.31,0.14,0]  InternalRulePriority=Speed  RndMeth=Simplest
  1-D Lookup Table2 : Lookup_n-D  NumberOfTableDimensions=1  BreakpointsForDimension1=[0,10,20,30,40,50,60,70,80,90]  Table=[0.04,0.04,0.04,0.04,0.05,0.05,0.08,0.175,0.38,1]  InternalRulePriority=Speed  RndMeth=Simplest
  1-D Lookup Table3 : Lookup_n-D  NumberOfTableDimensions=1  BreakpointsForDimension1=[0,10,20,30,40,50,60,70,80,90]  Table=[0.04,0.04,0.04,0.04,0.05,0.05,0.08,0.175,0.38,1]  InternalRulePriority=Speed  RndMeth=Simplest
  1-D Lookup Table4 : Lookup_n-D  NumberOfTableDimensions=1  BreakpointsForDimension1=[0,10,20,30,40,50,60,70,80,90]  Table=[0.43,0.435,0.44,0.45,0.455,0.48,0.505,0.515,0.48,0]  InternalRulePriority=Speed  RndMeth=Simplest
  1-D Lookup Table5 : Lookup_n-D  NumberOfTableDimensions=1  BreakpointsForDimension1=[0,10,20,30,40,50,60,70,80,90]  Table=[0.43,0.435,0.44,0.45,0.455,0.48,0.505,0.515,0.48,0]  InternalRulePriority=Speed  RndMeth=Simplest
  Add : Sum
  Add1 : Sum
  Add2 : Sum
  Constant : Constant  Value=180
  Constant1 : Constant  Value=180
  Constant2 : Constant  Value=180
  Fcn1 : Fcn  Expr=59.68-0.1457*u+0.001585*u^2
  Fcn2 : Fcn  Expr=59.68-0.1457*u+0.001585*u^2
  Fcn5 : Fcn  Expr=59.68-0.1457*u+0.001585*u^2
  Product1 : Product  Inputs=*/
  Product2 : Product
  Product3 : Product  Inputs=***
  Product4 : Product
  Product5 : Product  Inputs=*/
  Product6 : Product  Inputs=***
  Product7 : Product
  Product8 : Product  Inputs=***
  Product9 : Product  Inputs=*/
  Reflected portion not currently used : Terminator
  Sum : Sum  Inputs=|+-
  Sum1 : Sum  Inputs=|+-
  Sum2 : Sum  Inputs=|+-
  Out1 : Outport  VectorParamsAs1DForOutWhenUnconnected=off
  Out2 : Outport  Port=2  VectorParamsAs1DForOutWhenUnconnected=off
  wires:
  Product2/1 -> Add/1
  Fcn5/1 -> 1-D Lookup Table1/1
  Product3/1 -> Add/2
  In1/1 -> 1-D Lookup Table4/1, 1-D Lookup Table2/1, 1-D Lookup Table/1
  1-D Lookup Table1/1 -> Product3/1
  1-D Lookup Table/1 -> Product2/1
  Add/1 -> Out1/1
  Constant/1 -> Product1/2, Sum/1
  Sum/1 -> Product1/1
  Product1/1 -> Product3/3
  Product4/1 -> Add1/1
  1-D Lookup Table2/1 -> Product4/1
  In3/1 -> Product7/2, Product4/2, Product2/2
  Product5/1 -> Product6/3
  Constant1/1 -> Product5/2, Sum1/1
  1-D Lookup Table3/1 -> Product6/1
  Sum1/1 -> Product5/1
  Fcn1/1 -> 1-D Lookup Table3/1
  Product6/1 -> Add1/2
  Product7/1 -> Add2/1
  1-D Lookup Table4/1 -> Product7/1
  Product8/1 -> Add2/2
  Sum2/1 -> Product9/1
  Product9/1 -> Product8/3
  Constant2/1 -> Product9/2, Sum2/1
  In4/1 -> Product8/2, Product6/2, Product3/2
  1-D Lookup Table5/1 -> Product8/1
  Fcn2/1 -> 1-D Lookup Table5/1
  In2/1 -> Fcn1/1, Sum1/2, Fcn2/1, Sum2/2, Sum/2, Fcn5/1
  Add1/1 -> Reflected portion not currently used/1
  Add2/1 -> Out2/1

== system Final_EWASP_VC/Subsystem_Room3/Utility/Subsystem1/integrate deltat's with initial wall temps as initial condition ==
  In1 : Inport
  In2 : Inport  Port=2
  In3 : Inport  Port=3
  In4 : Inport  Port=4
  Constant : Constant  Value=2
  Constant1 : Constant
  Constant2 : Constant  Value=wallStartTempExt
  Discrete-Time Integrator : DiscreteIntegrator  InitialConditionSource=external  SampleTime=-1  ICPrevOutput=DiscIntNeverNeededParam  ICPrevScaledInput=DiscIntNeverNeededParam
  Discrete-Time Integrator1 : DiscreteIntegrator  InitialConditionSource=external  SampleTime=-1  ICPrevOutput=DiscIntNeverNeededParam  ICPrevScaledInput=DiscIntNeverNeededParam
  Discrete-Time Integrator2 : DiscreteIntegrator  InitialConditionSource=external  SampleTime=-1  ICPrevOutput=DiscIntNeverNeededParam  ICPrevScaledInput=DiscIntNeverNeededParam
  Display : Display
  Divide : Product  Inputs=*/
  Minus1 : Sum
  Minus2 : Sum  Inputs=+-
  Room Initial Temp Table : LookupNDDirect  NumberOfTableDimensions=1  Table=wallStartTempInt'
  Scope{,1..4} (5 alike) : Scope
  Out1 : Outport  VectorParamsAs1DForOutWhenUnconnected=off
  Out2 : Outport  Port=2  VectorParamsAs1DForOutWhenUnconnected=off
  Out3 : Outport  Port=3  VectorParamsAs1DForOutWhenUnconnected=off
  wires:
  Discrete-Time Integrator1/1 -> Scope1/1, Out2/1
  Discrete-Time Integrator2/1 -> Out1/1, Scope/1, Display/1
  Divide/1 -> Discrete-Time Integrator1/2
  In3/1 -> Discrete-Time Integrator/1
  Room Initial Temp Table/1 -> Discrete-Time Integrator2/2, Minus1/1, Scope3/1
  In2/1 -> Discrete-Time Integrator1/1
  Discrete-Time Integrator/1 -> Scope2/1, Out3/1
  Constant2/1 -> Discrete-Time Integrator/2, Minus1/2
  In1/1 -> Discrete-Time Integrator2/1
  In4/1 -> Scope4/1, Minus2/1
  Minus1/1 -> Divide/1
  Constant/1 -> Divide/2
  Constant1/1 -> Minus2/2
  Minus2/1 -> Room Initial Temp Table/1

== system Final_EWASP_VC/Subsystem_Room3/Utility/Subsystem3/integrate deltat's with initial wall temps as initial condition ==
  In1 : Inport
  In2 : Inport  Port=2
  In3 : Inport  Port=3
  In4 : Inport  Port=4
  Constant : Constant  Value=2
  Constant1 : Constant
  Constant2 : Constant  Value=wallStartTempExt
  Discrete-Time Integrator : DiscreteIntegrator  InitialConditionSource=external  SampleTime=-1  ICPrevOutput=DiscIntNeverNeededParam  ICPrevScaledInput=DiscIntNeverNeededParam
  Discrete-Time Integrator1 : DiscreteIntegrator  InitialConditionSource=external  SampleTime=-1  ICPrevOutput=DiscIntNeverNeededParam  ICPrevScaledInput=DiscIntNeverNeededParam
  Discrete-Time Integrator2 : DiscreteIntegrator  InitialConditionSource=external  SampleTime=-1  ICPrevOutput=DiscIntNeverNeededParam  ICPrevScaledInput=DiscIntNeverNeededParam
  Display : Display
  Divide : Product  Inputs=*/
  Minus1 : Sum
  Minus2 : Sum  Inputs=+-
  Room Initial Temp Table : LookupNDDirect  NumberOfTableDimensions=1  Table=roofStartTemp
  Scope{,1..2,4} (4 alike) : Scope
  Out1 : Outport  VectorParamsAs1DForOutWhenUnconnected=off
  Out2 : Outport  Port=2  VectorParamsAs1DForOutWhenUnconnected=off
  Out3 : Outport  Port=3  VectorParamsAs1DForOutWhenUnconnected=off
  wires:
  Discrete-Time Integrator1/1 -> Scope1/1, Out2/1
  Discrete-Time Integrator2/1 -> Out1/1, Scope/1, Display/1
  Divide/1 -> Discrete-Time Integrator1/2
  In3/1 -> Discrete-Time Integrator/1
  Room Initial Temp Table/1 -> Discrete-Time Integrator2/2, Minus1/1
  In2/1 -> Discrete-Time Integrator1/1
  Discrete-Time Integrator/1 -> Scope2/1, Out3/1
  Constant2/1 -> Discrete-Time Integrator/2, Minus1/2
  In1/1 -> Discrete-Time Integrator2/1
  In4/1 -> Scope4/1, Minus2/1
  Minus1/1 -> Divide/1
  Constant/1 -> Divide/2
  Constant1/1 -> Minus2/2
  Minus2/1 -> Room Initial Temp Table/1
